simulink model "Cinematique_ROS"  (R2020b)
settings: Solver=FixedStepDiscrete  StartTime=0.0  StopTime=inf  FixedStep=0.05  RelTol=1e-3
model workspace: external: MATLAB File C:\Users\antoi\OneDrive\Desktop\Matlab-Simulink\Test Robotique\Bras_DataFile.m (data not in the file)
libraries: robotlib x9, simulink x1, robotcorelib x1, robotmaniplib x1
settings Model: PacingRate=0.050000  Creator=antoi  LastModifiedBy=alessandrini
settings OptimizationCC: EnhancedBackFolding=on  PassReuseOutputArgsAs=Individual arguments  ZeroExternalMemoryAtStartup=off  ZeroInternalMemoryAtStartup=off  MaxStackSize=64  OptimizeBlockOrder=speed  DifferentSizesBufferReuse=on  OptimizationCustomize=off  EfficientTunableParamExpr=on
settings DebuggingCC: ParameterTunabilityLossMsg=error
settings HardwareCC: ProdBitPerPointer=32  ProdBitPerSizeT=32  ProdBitPerPtrDiffT=32  ProdLargestAtomicFloat=None  ProdIntDivRoundTo=Undefined  ProdEndianess=Unspecified  ProdWordSize=32  ProdHWDeviceType=Generic->Unspecified (assume 32-bit Generic)  UseEmbeddedCoderFeatures=off
settings RTWCC: Description=Embedded Coder  SystemTargetFile=ert.tlc  HardwareBoard=Robot Operating System (ROS)  TLCOptions="-aInlineSetEventsForThisBaseRateFcn=TLC_FALSE -aSuppressMultiTaskScheduler=TLC_FALSE  -aRateBasedStepFcn=0"  TemplateMakefile=ert_default_tmf  GenerateReport=on  Toolchain=Catkin  LaunchReport=on  TargetLang=C++
settings CodeAppCC: ForceParamTrailComments=on  IgnoreCustomStorageClasses=off  OperatorAnnotations=on  SimulinkDataObjDesc=on  SFDataObjDesc=on  InsertBlockDesc=on
settings ERTTargetCC: SupportNonInlinedSFcns=on

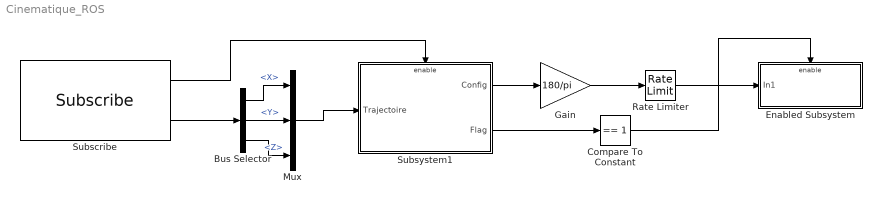
== system Cinematique_ROS ==
  Bus Selector : BusSelector  OutputSignals=X,Y,Z
  Compare To Constant : simulink/Logic and Bit Operations/Compare To Constant  relop===  const=1  OutDataTypeStr=boolean
  Enabled Subsystem : Subsystem  TreatAsAtomicUnit=on
  Gain : Gain  Gain=180/pi
  Mux : Mux  Inputs=3
  Rate Limiter : RateLimiter  RisingSlewLimit=20  FallingSlewLimit=-20
  Subscribe : robotlib/Subscribe  topicSource=Specify your own  topic=/Position  messageType=geometry_msgs/Point  SampleTime=-1  legacyBusStruct=off  messageQueueLength=1
  Subsystem1 : Subsystem
  wires:
  Subscribe/1 -> Subsystem1/Enable
  Subsystem1/1(Config) -> Gain/1
  Subscribe/2 -> Bus Selector/1
  Bus Selector/2 -> Mux/2  "<Y>"
  Bus Selector/1 -> Mux/1  "<X>"
  Bus Selector/3 -> Mux/3  "<Z>"
  Gain/1 -> Rate Limiter/1
  Subsystem1/2(Flag) -> Compare To Constant/1
  Compare To Constant/1 -> Enabled Subsystem/Enable
  Rate Limiter/1 -> Enabled Subsystem/1(In1)
  Mux/1 -> Subsystem1/1(Trajectoire)

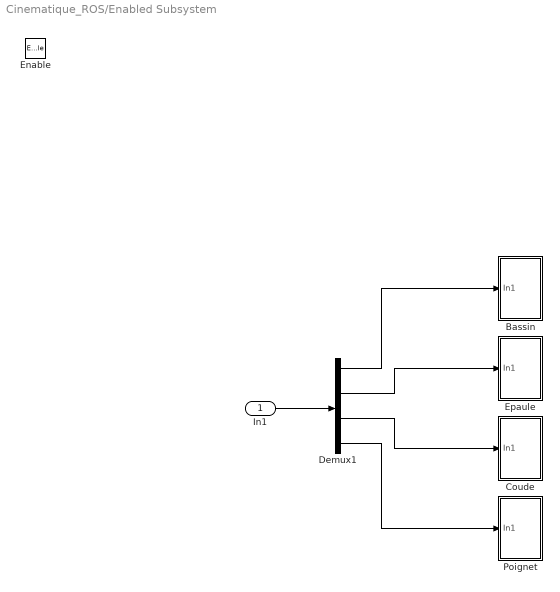
== system Cinematique_ROS/Enabled Subsystem ==
  In1 : Inport
  Enable : EnablePort
  Bassin : Subsystem
  Coude : Subsystem
  Demux1 : Demux
  Epaule : Subsystem
  Poignet : Subsystem
  wires:
  Demux1/2 -> Epaule/1(In1)
  Demux1/3 -> Coude/1(In1)
  In1/1 -> Demux1/1
  Demux1/1 -> Bassin/1(In1)
  Demux1/4 -> Poignet/1(In1)

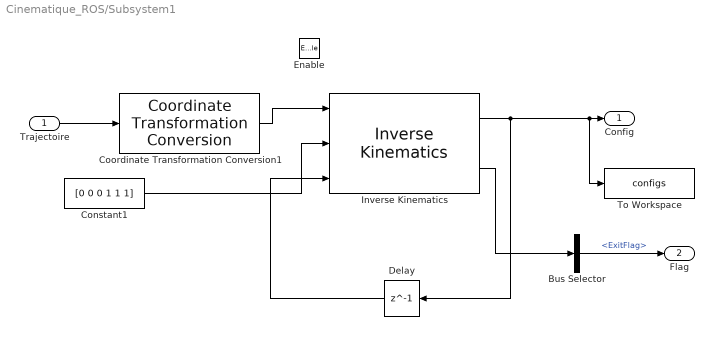
== system Cinematique_ROS/Subsystem1 ==
  Trajectoire : Inport
  Enable : EnablePort
  Bus Selector : BusSelector  OutputSignals=ExitFlag
  Constant1 : Constant  Value=[0 0 0 1 1 1]  VectorParams1D=off
  Coordinate Transformation Conversion1 : robotcorelib/Coordinate Transformation Conversion  InputRepresentation=Translation Vector  InputEulerSequence=ZYX  ShowTrVecInputPort=on  OutputRepresentation=Homogeneous Transformation  OutputEulerSequence=ZYX  ShowTrVecOutputPort=on  SimulateUsing=Interpreted execution
  Delay : Delay  DelayLength=1  InitialCondition=([90 140 -50 70]*pi/180)'
  Inverse Kinematics : robotmaniplib/Inverse Kinematics  RigidBodyTree=robot  EndEffector=Body5  ShowInfo=on  SolverName=BFGS Gradient Projection  EnforceJointLimits=on  MaxIterations=1500  MaxTime=10  GradientTolerance=1e-7  SolutionTolerance=1e-6  StepTolerance=1e-14  ErrorChangeTolerance=1e-12  UseErrorDamping=on  DampingBias=0.0025  SimulateUsing=Interpreted execution
  To Workspace : ToWorkspace  VariableName=configs  SaveFormat=Timeseries  SampleTime=-1
  Config : Outport
  Flag : Outport  Port=2
  wires:
  Coordinate Transformation Conversion1/1 -> Inverse Kinematics/1
  Inverse Kinematics/1 -> To Workspace/1, Config/1, Delay/1
  Delay/1 -> Inverse Kinematics/3
  Constant1/1 -> Inverse Kinematics/2
  Trajectoire/1 -> Coordinate Transformation Conversion1/1
  Inverse Kinematics/2 -> Bus Selector/1
  Bus Selector/1 -> Flag/1  "<ExitFlag>"

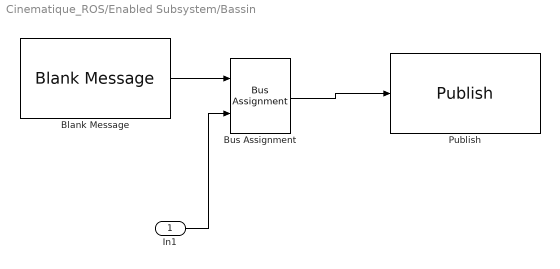
== system Cinematique_ROS/Enabled Subsystem/Bassin ==
  In1 : Inport
  Blank Message : robotlib/Blank Message  messageClass=Message  entityType=geometry_msgs/Point  messageType=geometry_msgs/Point  SampleTime=0.05  legacyBusStruct=off
  Bus Assignment : BusAssignment  AssignedSignals=X
  Publish : robotlib/Publish  topicSource=Specify your own  topic=/Bassin  messageType=geometry_msgs/Point  legacyBusStruct=off  messageQueueLength=1
  wires:
  Bus Assignment/1 -> Publish/1
  In1/1 -> Bus Assignment/2
  Blank Message/1 -> Bus Assignment/1

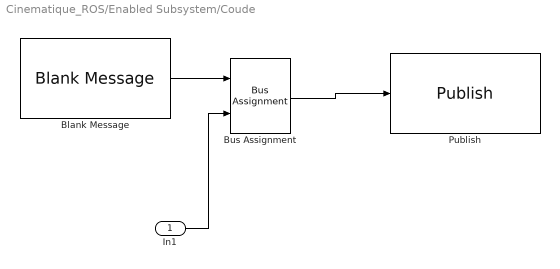
== system Cinematique_ROS/Enabled Subsystem/Coude ==
  In1 : Inport
  Blank Message : robotlib/Blank Message  messageClass=Message  entityType=geometry_msgs/Point  messageType=geometry_msgs/Point  SampleTime=0.05  legacyBusStruct=off
  Bus Assignment : BusAssignment  AssignedSignals=X
  Publish : robotlib/Publish  topicSource=Specify your own  topic=/Coude  messageType=geometry_msgs/Point  legacyBusStruct=off  messageQueueLength=1
  wires:
  Bus Assignment/1 -> Publish/1
  In1/1 -> Bus Assignment/2
  Blank Message/1 -> Bus Assignment/1

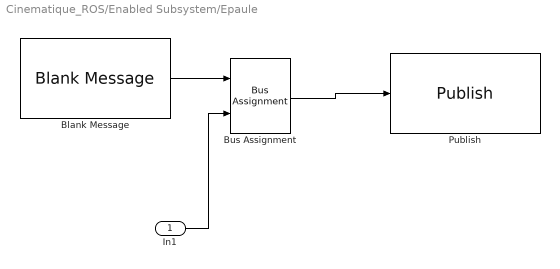
== system Cinematique_ROS/Enabled Subsystem/Epaule ==
  In1 : Inport
  Blank Message : robotlib/Blank Message  messageClass=Message  entityType=geometry_msgs/Point  messageType=geometry_msgs/Point  SampleTime=0.05  legacyBusStruct=off
  Bus Assignment : BusAssignment  AssignedSignals=X
  Publish : robotlib/Publish  topicSource=Specify your own  topic=/Epaule  messageType=geometry_msgs/Point  legacyBusStruct=off  messageQueueLength=1
  wires:
  Bus Assignment/1 -> Publish/1
  In1/1 -> Bus Assignment/2
  Blank Message/1 -> Bus Assignment/1

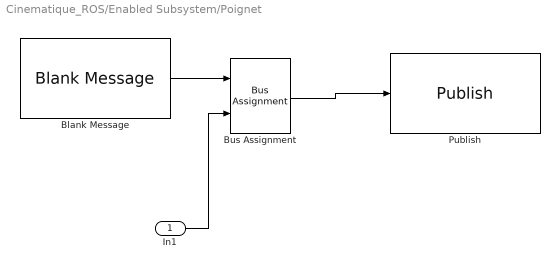
== system Cinematique_ROS/Enabled Subsystem/Poignet ==
  In1 : Inport
  Blank Message : robotlib/Blank Message  messageClass=Message  entityType=geometry_msgs/Point  messageType=geometry_msgs/Point  SampleTime=0.05  legacyBusStruct=off
  Bus Assignment : BusAssignment  AssignedSignals=X
  Publish : robotlib/Publish  topicSource=Specify your own  topic=/Poignet  messageType=geometry_msgs/Point  legacyBusStruct=off  messageQueueLength=1
  wires:
  Bus Assignment/1 -> Publish/1
  In1/1 -> Bus Assignment/2
  Blank Message/1 -> Bus Assignment/1
